simulink model "OpenLoopResponse"  (R2014a)
settings: Solver=ode45  StartTime=0.0  StopTime=10.0  RelTol=1e-3
settings Model: Creator=JATIN  LastModifiedBy=JATIN

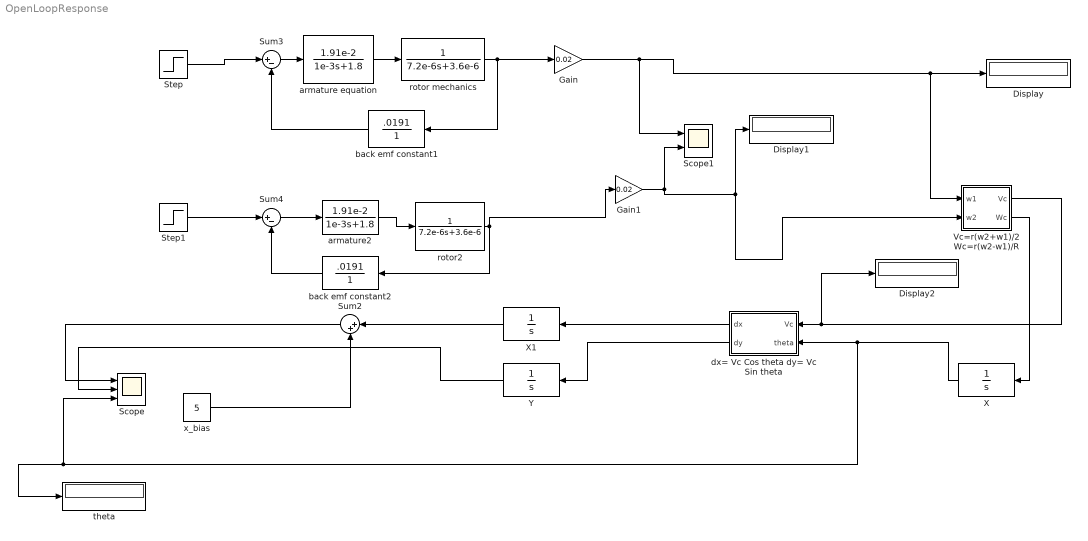
== system OpenLoopResponse ==
  Display : Display
  Display1 : Display
  Display2 : Display
  Gain : Gain  Gain=0.02
  Gain1 : Gain  Gain=0.02
  Scope : Scope  NumInputPorts=3
      settings: YMin=-5~-5~-5  YMax=5~5~5
  Scope1 : Scope  NumInputPorts=2
      settings: YMin=-5~-5  YMax=5~5
  Step : Step  Time=0  SampleTime=0
  Step1 : Step  Time=0  SampleTime=0
  Sum2 : Sum  Inputs=|++
  Sum3 : Sum  Inputs=|+-
  Sum4 : Sum  Inputs=|+-
  Vc=r(w2+w1)/2 Wc=r(w2-w1)/R : MATLAB Function  TreatAsAtomicUnit=on
  X : TransferFcn  Denominator=[1 0]
  X1 : TransferFcn  Denominator=[1 0]
  Y : TransferFcn  Denominator=[1 0]
  armature equation : TransferFcn  Numerator=[1.91e-2]  Denominator=[1e-3 1.8]
  armature2 : TransferFcn  Numerator=[1.91e-2]  Denominator=[1e-3 1.8]
  back emf constant1 : TransferFcn  Numerator=[.0191]  Denominator=[0 1]
  back emf constant2 : TransferFcn  Numerator=[.0191]  Denominator=[0 1]
  dx= Vc Cos theta dy= Vc Sin theta : MATLAB Function  TreatAsAtomicUnit=on
  rotor mechanics : TransferFcn  Denominator=[7.2e-6 3.6e-6]
  rotor2 : TransferFcn  Denominator=[7.2e-6 3.6e-6]
  theta : Display
  x_bias : Constant  Value=5
  wires:
  armature equation/1 -> rotor mechanics/1
  back emf constant1/1 -> Sum3/2
  Sum3/1 -> armature equation/1
  Sum4/1 -> armature2/1
  armature2/1 -> rotor2/1
  rotor2/1 -> Gain1/1, back emf constant2/1
  back emf constant2/1 -> Sum4/2
  Gain/1 -> Scope1/1, Display/1, Vc=r(w2+w1)/2 Wc=r(w2-w1)/R/1(w1)
  Gain1/1 -> Display1/1, Vc=r(w2+w1)/2 Wc=r(w2-w1)/R/2(w2), Scope1/2
  dx= Vc Cos theta dy= Vc Sin theta/2(dy) -> Y/1
  Vc=r(w2+w1)/2 Wc=r(w2-w1)/R/2(Wc) -> X/1
  rotor mechanics/1 -> back emf constant1/1, Gain/1
  Y/1 -> Scope/2
  dx= Vc Cos theta dy= Vc Sin theta/1(dx) -> X1/1
  Vc=r(w2+w1)/2 Wc=r(w2-w1)/R/1(Vc) -> Display2/1, dx= Vc Cos theta dy= Vc Sin theta/1(Vc)
  x_bias/1 -> Sum2/2
  Sum2/1 -> Scope/1
  X1/1 -> Sum2/1
  X/1 -> Scope/3, theta/1, dx= Vc Cos theta dy= Vc Sin theta/2(theta)
  Step/1 -> Sum3/1
  Step1/1 -> Sum4/1

== matlab function OpenLoopResponse/dx= Vc Cos theta dy= Vc Sin theta ==
  data: Vc input; theta input; dx output; dy output
function [dx,dy] = fcn(Vc,theta)
%#codegen
dx=Vc*cos(theta);
dy=Vc*sin(theta);

== matlab function OpenLoopResponse/Vc=r(w2+w1)//2 Wc=r(w2-w1)//R ==
  data: w1 input; Vc output; w2 input; Wc output
function [Vc,Wc] = fcn(w1,w2)
%#codegen
r = 0.0508;
R = 0.24;
Vc = r*(w2+w1)/2;
Wc = r*(w2-w1)/R;
